simulink subsystem "Piero_Controlado_Velocidad"  (R2023b)
settings: Solver=VariableStepAuto  StartTime=0.0  StopTime=10.0  RelTol=1e-3
settings Model: Creator=Enrique  LastModifiedBy=Enrique

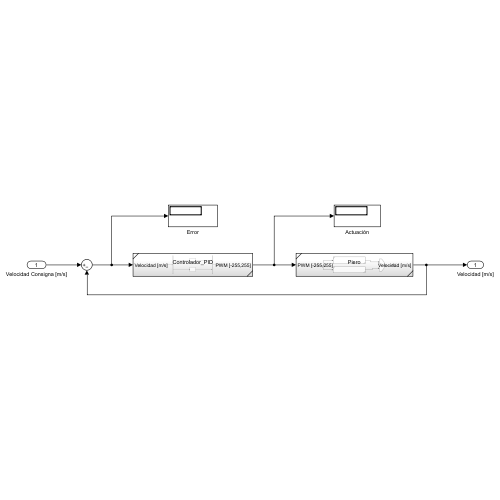
[thumbnail: Simulink's stored preview of the top-level diagram]
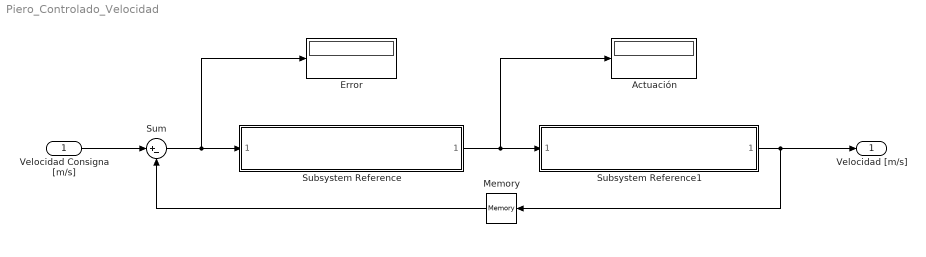
== system Piero_Controlado_Velocidad ==
  Velocidad Consigna [m/s] : Inport
  Actuación : Display
  Error : Display
  Memory : Memory
  Subsystem Reference : Subsystem  ReferencedSubsystem=Controlador_PID
  Subsystem Reference1 : Subsystem  ReferencedSubsystem=Piero
  Sum : Sum  Inputs=|+-
  Velocidad [m/s] : Outport
  wires:
  Velocidad Consigna [m/s]/1 -> Sum/1
  Subsystem Reference1/1 -> Velocidad [m/s]/1, Memory/1
  Subsystem Reference/1 -> Actuación/1, Subsystem Reference1/1
  Sum/1 -> Error/1, Subsystem Reference/1
  Memory/1 -> Sum/2
